simulink model "simple_lkas_mpc"  (R2017b)
settings: Solver=FixedStepAuto  StartTime=0.0  StopTime=15  FixedStep=0.1  RelTol=1e-3
values from neighbouring files (symbols this model uses):
  Cf = 19000    [mpc_lateral_control_data.mat]
  Iz = 2875    [mpc_lateral_control_data.mat]
  lf = 1.2    [mpc_lateral_control_data.mat]
  m = 1575    [mpc_lateral_control_data.mat]
  Ts = 0.1    [mpc_lateral_control_data.mat]
  Vx = 15    [mpc_lateral_control_data.mat]
libraries: mpclib x1
settings Model: Creator=nz82e7  LastModifiedBy=nz82e7

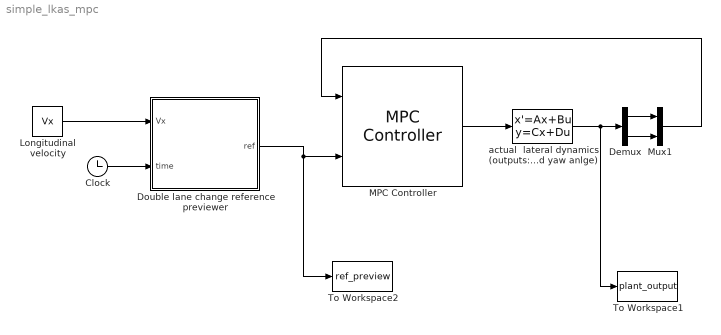
== system simple_lkas_mpc ==
  Clock : Clock
  Demux : Demux  Outputs=2
  "Double lane change reference previewer " : MATLAB Function  TreatAsAtomicUnit=on  SystemSampleTime=Ts
  Longitudinal velocity : Constant  Value=Vx  SampleTime=Ts
  MPC Controller : mpclib/MPC Controller  SCDEnableBlockLinearizationSpecification=on  mpcobj=mpc1  is_multiple=0  enable_value=0  return_u0=off  ref_from_ws=off  ref_signal_name=[]  ref_preview=off  md_from_ws=off  md_signal_name=[]  md_preview=off  from_project=off  project_file=MPCtask.mat  md_inport=off  mv_inport=off  cost_outport=off  return_sequence=off  return_qpstatus=off  return_state=off  state_inport=off  lims_inport=off  cc_inport=off  ywt_inport=off  is_designfromscratch=0  uwt_inport=off  duwt_inport=off  rhoeps_inport=off  uref_inport=off  n_ts=0.1  n_p=10  n_mv=1  n_md=0  n_ud=0  n_mo=2  n_uo=0  BlockDataType=double  SampleTimeInherited=off  switch_inport=off
  Mux1 : Mux  Inputs=2
  To Workspace1 : ToWorkspace  VariableName=plant_output  SaveFormat=Timeseries  SampleTime=-1
  To Workspace2 : ToWorkspace  VariableName=ref_preview  SaveFormat=Timeseries  SampleTime=-1
  actual  lateral dynamics (outputs: global Y and yaw anlge) : StateSpace  A=|  B=[2*Cf/m 0 2*Cf*lf/Iz 0]'  C=[0 0 0 1; 0 1 0 0]  D=[0;0]  InitialCondition=[0;0;0;0]
      | [-(2*Cf+2*Cr)/m/Vx, 0, -Vx-(2*Cf*lf-2*Cr*lr)/m/Vx, 0;
      |      0, 0, 1, 0;
      |      -(2*Cf*lf-2*Cr*lr)/Iz/Vx, 0, -(2*Cf*lf^2+2*Cr*lr^2)/Iz/Vx, 0;
      |      1, Vx, 0, 0]
  wires:
  MPC Controller/1 -> actual  lateral dynamics (outputs: global Y and yaw anlge)/1
  actual  lateral dynamics (outputs: global Y and yaw anlge)/1 -> To Workspace1/1, Demux/1
  Demux/1 -> Mux1/1
  Mux1/1 -> MPC Controller/1
  Demux/2 -> Mux1/2
  Longitudinal velocity/1 -> "Double lane change reference previewer "/1(Vx)
  Clock/1 -> "Double lane change reference previewer "/2(time)
  "Double lane change reference previewer "/1(ref) -> To Workspace2/1, MPC Controller/2

== matlab function simple_lkas_mpc/Double lane change reference previewer  ==
  data: Vx input; time input; ref output
function ref = previewer(Vx,time)
% Get previewed reference trajectory

% Previw horizon is 10 sampling times (i.e. 10*0.1 = 1 seconds).
% Reference contains 2 signals (i.e. Y position and yaw angle).
ref = zeros(10,2); 

%% Previewing sequence
for ct = 1:10
   [Yref,Zref,Xref] = doubleLaneChange(Vx,time + (ct-1)*0.1);
   ref(ct,1)=Yref;
   ref(ct,2)=Zref;
%    instant=time+(ct-1)*0.1;
%    if instant>5 && instant<10
%        ref(ct,1) = 1;
%        ref(ct,2) = 0; % Yaw angle can be done in a better way but mostly 0
%    else
%        ref(ct,1) = 0;
%        ref(ct,2) = 0;
%    end
end
